simulink model "BOX_JENKINS_SIMULINK_2"  (R2020b)
settings: Solver=FixedStepAuto  StartTime=0.0  StopTime=100  FixedStep=0.01  RelTol=1e-3
libraries: simulink x2
settings Model: Creator=alejandropuerta  LastModifiedBy=3.4b

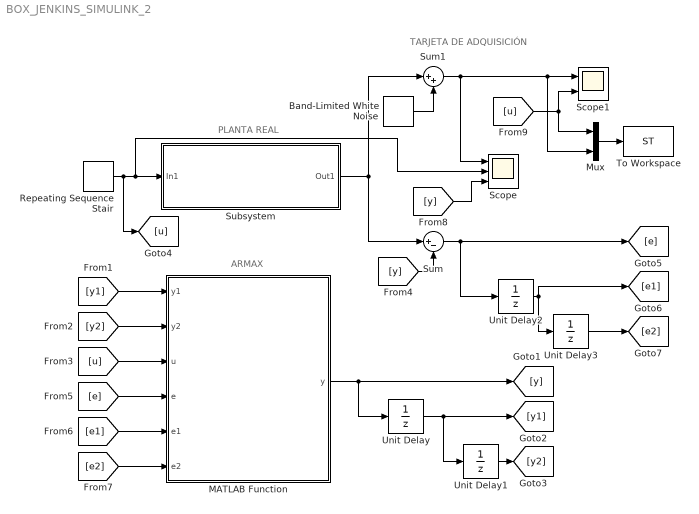
== system BOX_JENKINS_SIMULINK_2 ==
  note: TARJETA DE ADQUISICIÓN
  note: ARMAX
  note: PLANTA REAL
  Band-Limited White Noise : simulink/Sources/Band-Limited White Noise  Cov=[0.000001]  Ts=0.01  seed=[23341]
  MATLAB Function : MATLAB Function  TreatAsAtomicUnit=on
  Mux : Mux  Inputs=2
  Repeating Sequence Stair : simulink/Sources/Repeating Sequence Stair  OutValues=[0 0.2 0 0.4 0.8 0.4 1].'  tsamp=15  OutMin=[]  OutMax=[]  OutDataTypeStr=double  OutputDataTypeScalingMode=double  OutDataType=fixdt(0,8)  ConRadixGroup=Best Precision: Vector-wise  OutScaling=2^-12
  Scope : Scope  NumInputPorts=3
  Scope1 : Scope  NumInputPorts=2
  Subsystem : Subsystem
  Sum : Sum  Inputs=|+-
  Sum1 : Sum  Inputs=|++
  To Workspace : ToWorkspace  VariableName=ST  SampleTime=-1
      settings: Save2DSignal=2-D array (concatenate along first dimension)
  Unit Delay{,1..3} (4 alike) : UnitDelay  SampleTime=-1  HasFrameUpgradeWarning=on
  wires:
  Subsystem/1(Out1) -> Sum/1, Sum1/1
  Repeating Sequence Stair/1 -> [u], Scope/2, Subsystem/1(In1)
  MATLAB Function/1(y) -> [y], Unit Delay/1
  Unit Delay/1 -> [y1], Unit Delay1/1
  Unit Delay1/1 -> [y2]
  [y1] -> MATLAB Function/1(y1)
  [y2] -> MATLAB Function/2(y2)
  [u] -> MATLAB Function/3(u)
  [y] -> Sum/2
  Sum/1 -> Unit Delay2/1, [e]
  Unit Delay2/1 -> Unit Delay3/1, [e1]
  Unit Delay3/1 -> [e2]
  [e] -> MATLAB Function/4(e)
  [e1] -> MATLAB Function/5(e1)
  [e2] -> MATLAB Function/6(e2)
  [y] -> Scope/3
  Band-Limited White Noise/1 -> Sum1/2
  Sum1/1 -> Scope/1, Mux/2, Scope1/1
  Mux/1 -> To Workspace/1
  [u] -> Mux/1, Scope1/2

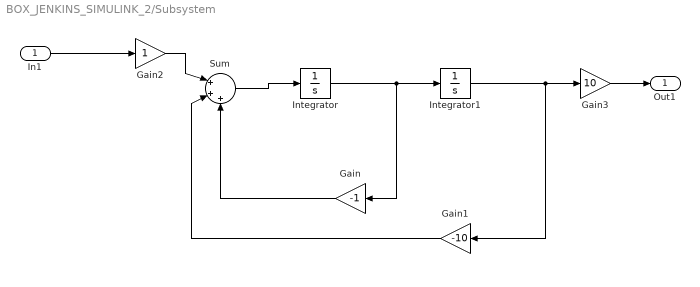
== system BOX_JENKINS_SIMULINK_2/Subsystem ==
  In1 : Inport
  Gain : Gain  Gain=-1
  Gain1 : Gain  Gain=-10
  Gain2 : Gain
  Gain3 : Gain  Gain=10
  Integrator : Integrator
  Integrator1 : Integrator
  Sum : Sum  Inputs=|+++
  Out1 : Outport  VectorParamsAs1DForOutWhenUnconnected=off
  wires:
  Integrator/1 -> Gain/1, Integrator1/1
  Gain2/1 -> Sum/1
  Gain1/1 -> Sum/2
  Sum/1 -> Integrator/1
  Integrator1/1 -> Gain3/1, Gain1/1
  Gain/1 -> Sum/3
  In1/1 -> Gain2/1
  Gain3/1 -> Out1/1

== matlab function BOX_JENKINS_SIMULINK_2/MATLAB Function ==
  data: y1 input; y2 input; u input; y output; e input; e1 input; e2 input
function y = fcn(y1,y2,u,e,e1,e2)

a1 = 1.989;
a2 = -0.99;
a3 = 0.0009799;
a4 = -1.967;
a5 = 0.9681;

y = a1*y1 + a2*y2 + a3*u + e + a4*e1 + a5*e2;
